simulink model "firefliesDemo"  (Simulink 7.4)
settings: Solver=ode3  StartTime=0.0  StopTime=200.0  FixedStep=0.5  RelTol=1e-3
values from neighbouring files (symbols this model uses):
  K = 0.1    [firefliesDemo.mat]
  N = 20    [firefliesDemo.mat]
  omega = 0.5    [firefliesDemo.mat]
  rho0 = 10    [firefliesDemo.mat]
  threshold = 4.71238898038    [firefliesDemo.mat]
  var = 10    [firefliesDemo.mat]
(part 2 of 2)

== system firefliesDemo/firefly9 ==
  In1 : Inport  OutDataType=fixdt(1, 16)  OutScaling=2^0
  In2 : Inport  Port=2
  In3 : Inport  Port=3
  In4 : Inport  Port=4
  In5 : Inport  Port=5
  In6 : Inport  Port=6
  In7 : Inport  Port=7
  In8 : Inport  Port=8
  In9 : Inport  Port=9
  In10 : Inport  Port=10
  In11 : Inport  Port=11
  In12 : Inport  Port=12
  In13 : Inport  Port=13
  In14 : Inport  Port=14
  In15 : Inport  Port=15
  In16 : Inport  Port=16
  In17 : Inport  Port=17
  In18 : Inport  Port=18
  In19 : Inport  Port=19
  In20 : Inport  Port=20
  Add : Sum  OutDataType=fixdt(1, 16)  OutScaling=2^-10
  Add1 : Sum  Inputs=+-  OutDataType=fixdt(1, 16)  OutScaling=2^-10
  Gain : Gain  Gain=K/N  ParameterDataType=fixdt(1, 16)  ParameterScaling=2^0  OutDataType=fixdt(1, 16)  OutScaling=2^0
  Integrator : Integrator  InitialConditionSource=external
  Mux : Mux  Inputs=20
  Scope : Scope
  Scope1 : Scope
  Sum of Elements : Sum  Inputs=+  OutDataType=fixdt(1, 16)  OutScaling=2^-10
  Threshold : Constant  Value=threshold  OutDataType=fixdt(1, 16)  OutScaling=2^0
  Trigonometric Function : Trigonometry
  angle speed : Constant  Value=omega  OutDataType=fixdt(1, 16)  OutScaling=2^0
  flash : Stateflow chart
  rho0 : Constant  Value=rho0+rand(1)*var  OutDataType=fixdt(1, 16)  OutScaling=2^0
  Out1 : Outport  OutDataType=fixdt(1, 16)  OutScaling=2^0
  wires:
  In20/1 -> Mux/20
  In19/1 -> Mux/19
  In18/1 -> Mux/18
  In17/1 -> Mux/17
  In16/1 -> Mux/16
  In15/1 -> Mux/15
  In14/1 -> Mux/14
  In13/1 -> Mux/13
  In12/1 -> Mux/12
  In11/1 -> Mux/11
  In10/1 -> Mux/10
  In9/1 -> Mux/9
  In8/1 -> Mux/8
  In7/1 -> Mux/7
  In6/1 -> Mux/6
  In5/1 -> Mux/5
  In4/1 -> Mux/4
  In3/1 -> Mux/3
  In2/1 -> Mux/2
  rho0/1 -> Integrator/2
  Threshold/1 -> flash/2(t)
  Sum of Elements/1 -> Gain/1
  Trigonometric Function/1 -> Sum of Elements/1
  Add/1 -> Scope1/1, flash/1(u), Integrator/1  "drho/dt"
  Gain/1 -> Add/2
  angle speed/1 -> Add/1
  Add1/1 -> Trigonometric Function/1
  Integrator/1 -> Scope/1, Out1/1, Add1/2  "rho_i"
  Mux/1 -> Add1/1
  In1/1 -> Mux/1

== matlab function firefly1/flash ==
  data: u input double; y output double; t input double
function y = fcn(u,t)
%#eml
% Allows the flashing of the subsystem block after some threshold
eml.extrinsic('set_param','get_param','gcs');

y = u;

if u > t
set_param(get_param(gcs,'parent'),'BackgroundColor','[0.3, 0.9, 0.5]');
else
set_param(get_param(gcs,'parent'),'BackgroundColor','white');
end

y = u;

== matlab function firefly/flash ==
  data: u input double; y output double; t input double
function y = fcn(u,t)
%#eml
% Allows the flashing of the subsystem block after some threshold
eml.extrinsic('set_param','get_param','gcs');

y = u;

if u > t
set_param(get_param(gcs,'parent'),'BackgroundColor','[0.3, 0.9, 0.5]');
else
set_param(get_param(gcs,'parent'),'BackgroundColor','white');
end

y = u;

== matlab function firefly2/flash ==
  data: u input double; y output double; t input double
function y = fcn(u,t)
%#eml
% Allows the flashing of the subsystem block after some threshold
eml.extrinsic('set_param','get_param','gcs');

y = u;

if u > t
set_param(get_param(gcs,'parent'),'BackgroundColor','[0.3, 0.9, 0.5]');
else
set_param(get_param(gcs,'parent'),'BackgroundColor','white');
end

y = u;

== matlab function firefly3/flash ==
  data: u input double; y output double; t input double
function y = fcn(u,t)
%#eml
% Allows the flashing of the subsystem block after some threshold
eml.extrinsic('set_param','get_param','gcs');

y = u;

if u > t
set_param(get_param(gcs,'parent'),'BackgroundColor','[0.3, 0.9, 0.5]');
else
set_param(get_param(gcs,'parent'),'BackgroundColor','white');
end

y = u;

== matlab function firefly4/flash ==
  data: u input double; y output double; t input double
function y = fcn(u,t)
%#eml
% Allows the flashing of the subsystem block after some threshold
eml.extrinsic('set_param','get_param','gcs');

y = u;

if u > t
set_param(get_param(gcs,'parent'),'BackgroundColor','[0.3, 0.9, 0.5]');
else
set_param(get_param(gcs,'parent'),'BackgroundColor','white');
end

y = u;

== matlab function firefly5/flash ==
  data: u input double; y output double; t input double
function y = fcn(u,t)
%#eml
% Allows the flashing of the subsystem block after some threshold
eml.extrinsic('set_param','get_param','gcs');

y = u;

if u > t
set_param(get_param(gcs,'parent'),'BackgroundColor','[0.3, 0.9, 0.5]');
else
set_param(get_param(gcs,'parent'),'BackgroundColor','white');
end

y = u;

== matlab function firefly6/flash ==
  data: u input double; y output double; t input double
function y = fcn(u,t)
%#eml
% Allows the flashing of the subsystem block after some threshold
eml.extrinsic('set_param','get_param','gcs');

y = u;

if u > t
set_param(get_param(gcs,'parent'),'BackgroundColor','[0.3, 0.9, 0.5]');
else
set_param(get_param(gcs,'parent'),'BackgroundColor','white');
end

y = u;

== matlab function firefly7/flash ==
  data: u input double; y output double; t input double
function y = fcn(u,t)
%#eml
% Allows the flashing of the subsystem block after some threshold
eml.extrinsic('set_param','get_param','gcs');

y = u;

if u > t
set_param(get_param(gcs,'parent'),'BackgroundColor','[0.3, 0.9, 0.5]');
else
set_param(get_param(gcs,'parent'),'BackgroundColor','white');
end

y = u;

== matlab function firefly8/flash ==
  data: u input double; y output double; t input double
function y = fcn(u,t)
%#eml
% Allows the flashing of the subsystem block after some threshold
eml.extrinsic('set_param','get_param','gcs');

y = u;

if u > t
set_param(get_param(gcs,'parent'),'BackgroundColor','[0.3, 0.9, 0.5]');
else
set_param(get_param(gcs,'parent'),'BackgroundColor','white');
end

y = u;

== matlab function firefly9/flash ==
  data: u input double; y output double; t input double
function y = fcn(u,t)
%#eml
% Allows the flashing of the subsystem block after some threshold
eml.extrinsic('set_param','get_param','gcs');

y = u;

if u > t
set_param(get_param(gcs,'parent'),'BackgroundColor','[0.3, 0.9, 0.5]');
else
set_param(get_param(gcs,'parent'),'BackgroundColor','white');
end

y = u;

== matlab function firefly10/flash ==
  data: u input double; y output double; t input double
function y = fcn(u,t)
%#eml
% Allows the flashing of the subsystem block after some threshold
eml.extrinsic('set_param','get_param','gcs');

y = u;

if u > t
set_param(get_param(gcs,'parent'),'BackgroundColor','[0.3, 0.9, 0.5]');
else
set_param(get_param(gcs,'parent'),'BackgroundColor','white');
end

y = u;

== matlab function firefly11/flash ==
  data: u input double; y output double; t input double
function y = fcn(u,t)
%#eml
% Allows the flashing of the subsystem block after some threshold
eml.extrinsic('set_param','get_param','gcs');

y = u;

if u > t
set_param(get_param(gcs,'parent'),'BackgroundColor','[0.3, 0.9, 0.5]');
else
set_param(get_param(gcs,'parent'),'BackgroundColor','white');
end

y = u;

== matlab function firefly12/flash ==
  data: u input double; y output double; t input double
function y = fcn(u,t)
%#eml
% Allows the flashing of the subsystem block after some threshold
eml.extrinsic('set_param','get_param','gcs');

y = u;

if u > t
set_param(get_param(gcs,'parent'),'BackgroundColor','[0.3, 0.9, 0.5]');
else
set_param(get_param(gcs,'parent'),'BackgroundColor','white');
end

y = u;

== matlab function firefly13/flash ==
  data: u input double; y output double; t input double
function y = fcn(u,t)
%#eml
% Allows the flashing of the subsystem block after some threshold
eml.extrinsic('set_param','get_param','gcs');

y = u;

if u > t
set_param(get_param(gcs,'parent'),'BackgroundColor','[0.3, 0.9, 0.5]');
else
set_param(get_param(gcs,'parent'),'BackgroundColor','white');
end

y = u;

== matlab function firefly14/flash ==
  data: u input double; y output double; t input double
function y = fcn(u,t)
%#eml
% Allows the flashing of the subsystem block after some threshold
eml.extrinsic('set_param','get_param','gcs');

y = u;

if u > t
set_param(get_param(gcs,'parent'),'BackgroundColor','[0.3, 0.9, 0.5]');
else
set_param(get_param(gcs,'parent'),'BackgroundColor','white');
end

y = u;

== matlab function firefly15/flash ==
  data: u input double; y output double; t input double
function y = fcn(u,t)
%#eml
% Allows the flashing of the subsystem block after some threshold
eml.extrinsic('set_param','get_param','gcs');

y = u;

if u > t
set_param(get_param(gcs,'parent'),'BackgroundColor','[0.3, 0.9, 0.5]');
else
set_param(get_param(gcs,'parent'),'BackgroundColor','white');
end

y = u;

== matlab function firefly16/flash ==
  data: u input double; y output double; t input double
function y = fcn(u,t)
%#eml
% Allows the flashing of the subsystem block after some threshold
eml.extrinsic('set_param','get_param','gcs');

y = u;

if u > t
set_param(get_param(gcs,'parent'),'BackgroundColor','[0.3, 0.9, 0.5]');
else
set_param(get_param(gcs,'parent'),'BackgroundColor','white');
end

y = u;

== matlab function firefly17/flash ==
  data: u input double; y output double; t input double
function y = fcn(u,t)
%#eml
% Allows the flashing of the subsystem block after some threshold
eml.extrinsic('set_param','get_param','gcs');

y = u;

if u > t
set_param(get_param(gcs,'parent'),'BackgroundColor','[0.3, 0.9, 0.5]');
else
set_param(get_param(gcs,'parent'),'BackgroundColor','white');
end

y = u;

== matlab function firefly18/flash ==
  data: u input double; y output double; t input double
function y = fcn(u,t)
%#eml
% Allows the flashing of the subsystem block after some threshold
eml.extrinsic('set_param','get_param','gcs');

y = u;

if u > t
set_param(get_param(gcs,'parent'),'BackgroundColor','[0.3, 0.9, 0.5]');
else
set_param(get_param(gcs,'parent'),'BackgroundColor','white');
end

y = u;

== matlab function firefly19/flash ==
  data: u input double; y output double; t input double
function y = fcn(u,t)
%#eml
% Allows the flashing of the subsystem block after some threshold
eml.extrinsic('set_param','get_param','gcs');

y = u;

if u > t
set_param(get_param(gcs,'parent'),'BackgroundColor','[0.3, 0.9, 0.5]');
else
set_param(get_param(gcs,'parent'),'BackgroundColor','white');
end

y = u;
